simulink model "mcb_pmsm_foc_host_model_f28379d"  (R2023b)
settings: Solver=FixedStepDiscrete  StartTime=0.0  StopTime=inf  RelTol=1e-3  EnableMultiTasking=on
values from neighbouring files (symbols this model uses):
  dataType = 'single'    [mcb_pmsm_foc_sensorless_f28379d_datascript.m]    (also in mcb_pmsm_foc_test_f28379d_data.m)
  PU_System = mcb_SetPUSystem(pmsm,inverter)    [mcb_pmsm_foc_sensorless_f28379d_datascript.m]    (also in mcb_pmsm_foc_test_f28379d_data.m)
  Ts = T_pwm    [discrete_tansfer_fcn.m]    (also in mcb_pmsm_foc_sensorless_f28379d_datascript.m = 5e-05; mcb_pmsm_foc_test_f28379d_data.m = 5e-05)
libraries: instrumentseriallib x4, simulink x3
settings Model: Creator=The MathWorks, Inc.  LastModifiedBy=13571
settings SolverCC: AlgebraicLoopSolver=TrustRegion  MaxZcPerStep=1
settings DataIOCC: LimitDataPoints=on  SaveFormat=Array  ReturnWorkspaceOutputs=off
settings OptimizationCC: ReuseModelBlockBuffer=off  LifeSpan=1  EfficientTunableParamExpr=on
settings DebuggingCC: UnderspecifiedInitializationDetection=Classic  MergeDetectMultiDrivingBlocksExec=none  SolverPrmCheckMsg=warning  ParameterPrecisionLossMsg=none  UnconnectedInputMsg=warning  UnconnectedOutputMsg=warning  UnconnectedLineMsg=warning  AllowSymbolicDim=off  PregeneratedLibrarySubsystemCodeDiagnostic=none  SFUnexpectedBacktrackingDiag=warning  SFNoUnconditionalDefaultTransitionDiag=warning  SFExecutionAtInitializationDiag=none  ArithmeticOperatorsInVariantConditions=warning
settings HardwareCC: ProdBitPerPointer=32  ProdLargestAtomicFloat=None  ProdIntDivRoundTo=Undefined  ProdEndianess=Unspecified  ProdWordSize=32  ProdHWDeviceType=32-bit Generic
settings ModelReferenceCC: EnableRefExpFcnMdlSchedulingChecks=on  PropagateSignalLabelsOutOfModel=off
settings SFSimCC: SimUseLocalCustomCode=off  MATLABDynamicMemAlloc=off
settings RTWCC: Description=Real-Time Workshop Embedded Coder  SystemTargetFile=ert.tlc  TemplateMakefile=ert_default_tmf  GenerateReport=on  RTWUseLocalCustomCode=off  IncludeHyperlinkInReport=on  LaunchReport=on  GenerateTraceInfo=on  GenerateTraceReport=on  GenerateTraceReportSl=on  GenerateTraceReportSf=on  GenerateTraceReportEml=on  DLArmComputeVersion=19.05
settings CodeAppCC: IgnoreCustomStorageClasses=off  StateflowObjectComments=on  InternalIdentifier=Classic
settings ERTTargetCC: MultiwordLength=2048  GenerateSampleERTMain=on  ERTCustomFileTemplate=example_file_process.tlc  ConvertIfToSwitch=off  SuppressUnreachableDefaultCases=off
settings ConfigComp: CovMetricSettings=dw  CovSaveCumulativeToWorkspaceVar=on  CovSaveSingleToWorkspaceVar=on  CovExternalEMLEnable=off  CovSFcnEnable=off

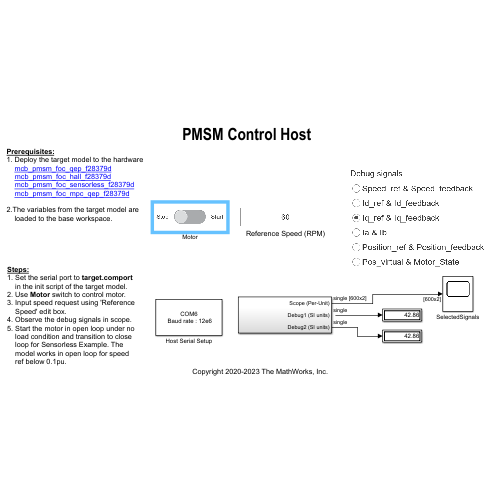
[thumbnail: Simulink's stored preview of the top-level diagram]
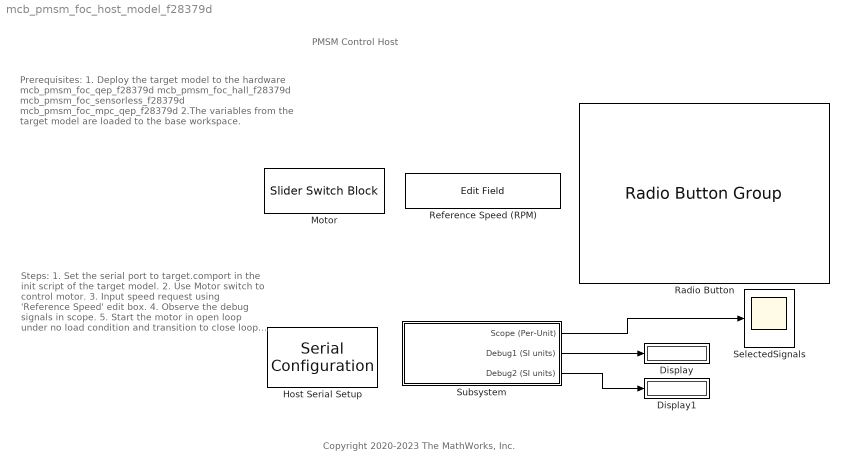
== system mcb_pmsm_foc_host_model_f28379d ==
  note: PMSM Control Host
  note: Copyright 2020-2023 The MathWorks, Inc.
  note: Steps:
      | 1. Set the serial port to target.comport
      | in the init script of the target model.
      | 2. Use Motor switch to control motor.
      | 3. Input speed request using 'Reference
      | Speed' edit box.
      | 4. Observe the debug signals in scope.
      | 5. Start the motor in open loop under no
      | load condition and transition to close
      | loop for Sensorless Example. The
      | model works in open loop for speed
      | ref below 0.1pu.
  note: Prerequisites:
      | 1. Deploy the target model to the hardware
      | mcb_pmsm_foc_qep_f28379d
      | mcb_pmsm_foc_hall_f28379d
      | mcb_pmsm_foc_sensorless_f28379d
      | mcb_pmsm_foc_mpc_qep_f28379d
      |
      | 2.The variables from the target model are
      | loaded to the base workspace.
  Display : Display
  Display1 : Display
  Host Serial Setup : instrumentseriallib/Serial Configuration  Priority=-99  PortSel=COM6  Port=COM6  ComPort=COM6  BaudRate=12e6  DataBits=8  Parity=none  StopBits=1  ByteOrder=little-endian  FlowControl=none  Timeout=2  SimulateUsing=Interpreted execution  BlockInModel=on  aMode=5
  Motor : SliderSwitchBlock  LabelPosition=Hide
      settings: Values={{'Stop', 'Start'}, [0 1]}
  Radio Button : RadioButtonGroup  LabelPosition=Hide  SelectedLabel=Iq_ref & Iq_feedback  ButtonGroupName=Debug signals
      settings: Values={{'Speed_ref & Speed_feedback', 'Id_ref & Id_feedback', 'Iq_ref & Iq_feedback', 'Ia & Ib', 'Position_ref & Position_feedback', 'Pos_virtual & Motor_State'}, [1 2 3 4 5 6]}
  Reference Speed (RPM) : EditField  LabelPosition=Hide  ShowInitialText=on  Alignment=Center
  SelectedSignals : Scope
  Subsystem : Subsystem
  wires:
  Subsystem/1(Scope (Per-Unit)) -> SelectedSignals/1
  Subsystem/2(Debug1 (SI units)) -> Display/1
  Subsystem/3(Debug2 (SI units)) -> Display1/1

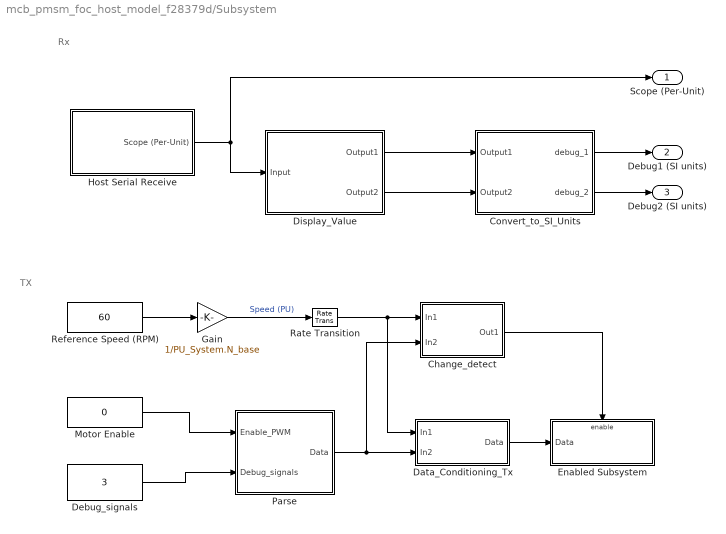
== system mcb_pmsm_foc_host_model_f28379d/Subsystem ==
  note: Rx
  note: TX
  Change_detect : Subsystem
  Convert_to_SI_Units : Subsystem
  Data_Conditioning_Tx : Subsystem  Variant=on
  Debug_signals : Constant  Value=3  OutDataTypeStr=uint16  SampleTime=0.03
  Display_Value : MATLAB Function  TreatAsAtomicUnit=on
  Enabled Subsystem : Subsystem  TreatAsAtomicUnit=on
  Gain : Gain  Gain=1/PU_System.N_base  RndMeth=Simplest  OutDataTypeStr=Inherit: Same as input
  Host Serial Receive : Subsystem  Variant=on
  Motor Enable : Constant  Value=0  VectorParams1D=off  OutDataTypeStr=uint16  SampleTime=0.03
  Parse : Subsystem
  Rate Transition : RateTransition  OutPortSampleTime=0.03
  Reference Speed (RPM) : Constant  Value=60  VectorParams1D=off  OutDataTypeStr=single  SampleTime=0.03
  Scope (Per-Unit) : Outport
  Debug1 (SI units) : Outport  Port=2
  Debug2 (SI units) : Outport  Port=3
  wires:
  Motor Enable/1 -> Parse/1(Enable_PWM)
  Change_detect/1(Out1) -> Enabled Subsystem/Enable
  Reference Speed (RPM)/1 -> Gain/1
  Rate Transition/1 -> Data_Conditioning_Tx/1(In1), Change_detect/1(In1)
  Parse/1(Data) -> Data_Conditioning_Tx/2(In2), Change_detect/2(In2)
  Data_Conditioning_Tx/1(Data) -> Enabled Subsystem/1(Data)
  Gain/1 -> Rate Transition/1  "Speed (PU)"
  Debug_signals/1 -> Parse/2(Debug_signals)
  Display_Value/2(Output2) -> Convert_to_SI_Units/2(Output2)
  Display_Value/1(Output1) -> Convert_to_SI_Units/1(Output1)
  Convert_to_SI_Units/2(debug_2) -> Debug2 (SI units)/1
  Convert_to_SI_Units/1(debug_1) -> Debug1 (SI units)/1
  Host Serial Receive/1(Scope (Per-Unit)) -> Scope (Per-Unit)/1, Display_Value/1(Input)

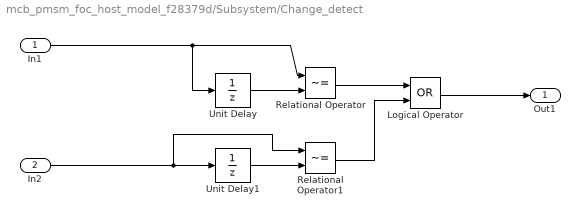
== system mcb_pmsm_foc_host_model_f28379d/Subsystem/Change_detect ==
  In1 : Inport
  In2 : Inport  Port=2
  Logical Operator : Logic  Operator=OR  AllPortsSameDT=off  OutDataTypeStr=boolean
  Relational Operator : RelationalOperator  Operator=~=  OutDataTypeStr=boolean  InputSameDT=off
  Relational Operator1 : RelationalOperator  Operator=~=  OutDataTypeStr=boolean  InputSameDT=off
  Unit Delay : UnitDelay  InitialCondition=0.5  SampleTime=-1  HasFrameUpgradeWarning=on
  Unit Delay1 : UnitDelay  SampleTime=-1  HasFrameUpgradeWarning=on
  Out1 : Outport  VectorParamsAs1DForOutWhenUnconnected=off
  wires:
  In2/1 -> Relational Operator1/1, Unit Delay1/1
  Relational Operator1/1 -> Logical Operator/2
  Unit Delay1/1 -> Relational Operator1/2
  Unit Delay/1 -> Relational Operator/2
  In1/1 -> Unit Delay/1, Relational Operator/1
  Relational Operator/1 -> Logical Operator/1
  Logical Operator/1 -> Out1/1

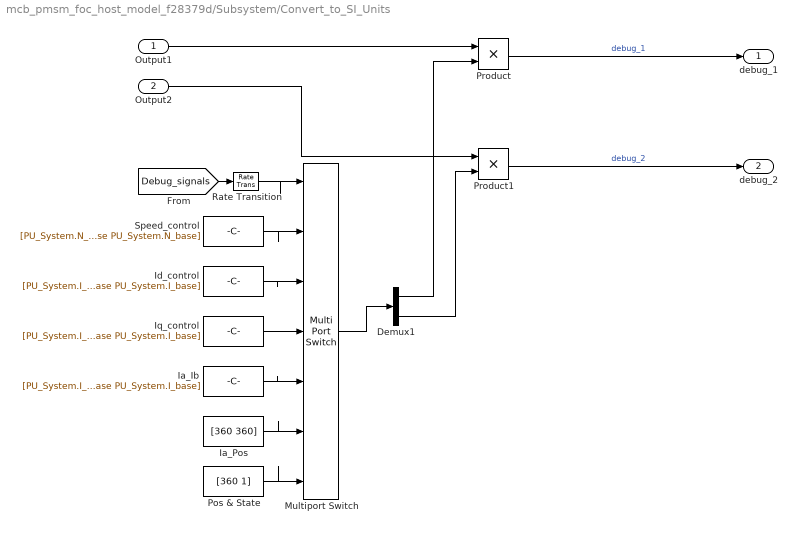
== system mcb_pmsm_foc_host_model_f28379d/Subsystem/Convert_to_SI_Units ==
  Output1 : Inport
  Output2 : Inport  Port=2
  Demux1 : Demux  Outputs=2
  Ia_Ib : Constant  Value=[PU_System.I_base PU_System.I_base]  OutDataTypeStr=single  SampleTime=-1
  Ia_Pos : Constant  Value=[360 360]  OutDataTypeStr=single  SampleTime=-1
  Id_control : Constant  Value=[PU_System.I_base PU_System.I_base]  OutDataTypeStr=single  SampleTime=-1
  Iq_control : Constant  Value=[PU_System.I_base PU_System.I_base]  OutDataTypeStr=single  SampleTime=-1
  Multiport Switch : MultiPortSwitch  Inputs=6  DiagnosticForDefault=Warning  OutDataTypeStr=single  RndMeth=Simplest  SaturateOnIntegerOverflow=off  InputSameDT=off
  Pos & State : Constant  Value=[360 1]  OutDataTypeStr=single  SampleTime=-1
  Product : Product
  Product1 : Product
  Rate Transition : RateTransition  Deterministic=off
  Speed_control : Constant  Value=[PU_System.N_base PU_System.N_base]  OutDataTypeStr=single  SampleTime=-1
  debug_1 : Outport
  debug_2 : Outport  Port=2
  wires:
  Product/1 -> debug_1/1  "debug_1"
  Product1/1 -> debug_2/1  "debug_2"
  [Debug_signals] -> Rate Transition/1
  Id_control/1 -> Multiport Switch/3
  Speed_control/1 -> Multiport Switch/2
  Multiport Switch/1 -> Demux1/1
  Ia_Ib/1 -> Multiport Switch/5
  Iq_control/1 -> Multiport Switch/4
  Demux1/2 -> Product1/2
  Demux1/1 -> Product/2
  Ia_Pos/1 -> Multiport Switch/6
  Output1/1 -> Product/1
  Output2/1 -> Product1/1
  Rate Transition/1 -> Multiport Switch/1
  Pos & State/1 -> Multiport Switch/7

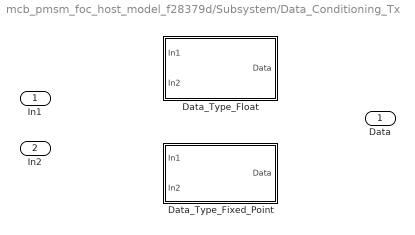
== system mcb_pmsm_foc_host_model_f28379d/Subsystem/Data_Conditioning_Tx ==
  In1 : Inport
  In2 : Inport  Port=2
  Data_Type_Fixed_Point : Subsystem  VariantControl=~isequal(dataType, 'single')
  Data_Type_Float : Subsystem  VariantControl=isequal(dataType, 'single')
  Data : Outport

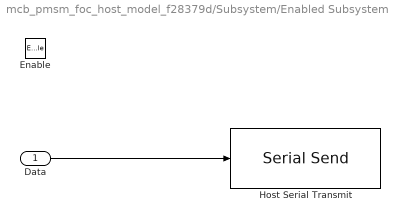
== system mcb_pmsm_foc_host_model_f28379d/Subsystem/Enabled Subsystem ==
  Data : Inport
  Enable : EnablePort
  Host Serial Transmit : instrumentseriallib/Serial Send  PortSel=COM6  Port=COM6  ComPort=COM6  Header=[]  Terminator=<none>  CustomTerminator=[]  EnableBlockingMode=off  SimulateUsing=Interpreted execution  BlockInModel=on  aMode=5
  wires:
  Data/1 -> Host Serial Transmit/1

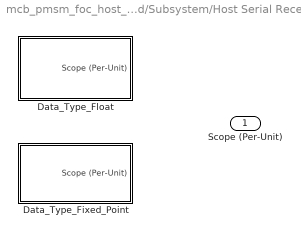
== system mcb_pmsm_foc_host_model_f28379d/Subsystem/Host Serial Receive ==
  Data_Type_Fixed_Point : Subsystem  VariantControl=~isequal(dataType, 'single')
  Data_Type_Float : Subsystem  VariantControl=isequal(dataType, 'single')
  Scope (Per-Unit) : Outport

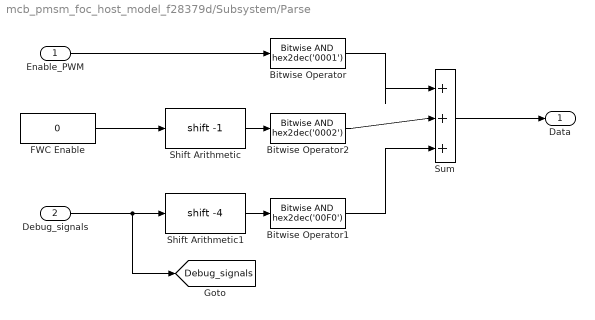
== system mcb_pmsm_foc_host_model_f28379d/Subsystem/Parse ==
  Enable_PWM : Inport
  Debug_signals : Inport  Port=2
  Bitwise Operator : simulink/Logic and Bit Operations/Bitwise Operator  logicop=AND  UseBitMask=on  BitMask=hex2dec('0001')  BitMaskRealWorld=Stored Integer
  Bitwise Operator1 : simulink/Logic and Bit Operations/Bitwise Operator  logicop=AND  UseBitMask=on  BitMask=hex2dec('00F0')  BitMaskRealWorld=Stored Integer
  Bitwise Operator2 : simulink/Logic and Bit Operations/Bitwise Operator  logicop=AND  UseBitMask=on  BitMask=hex2dec('0002')  BitMaskRealWorld=Stored Integer
  FWC Enable : Constant  Value=0  VectorParams1D=off  OutDataTypeStr=uint16  SampleTime=0.03
  Shift Arithmetic : ArithShift  BitShiftNumber=-1
  Shift Arithmetic1 : ArithShift  BitShiftNumber=-4
  Sum : Sum  Inputs=|+++
  Data : Outport
  tag scope: Debug_signals=global
  wires:
  Bitwise Operator/1 -> Sum/1
  Debug_signals/1 -> [Debug_signals], Shift Arithmetic1/1
  Sum/1 -> Data/1
  Shift Arithmetic1/1 -> Bitwise Operator1/1
  Shift Arithmetic/1 -> Bitwise Operator2/1
  Bitwise Operator1/1 -> Sum/3
  FWC Enable/1 -> Shift Arithmetic/1
  Bitwise Operator2/1 -> Sum/2
  Enable_PWM/1 -> Bitwise Operator/1

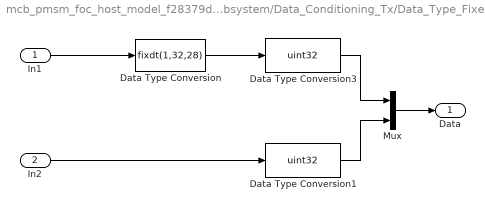
== system mcb_pmsm_foc_host_model_f28379d/Subsystem/Data_Conditioning_Tx/Data_Type_Fixed_Point ==
  In1 : Inport
  In2 : Inport  Port=2
  Data Type Conversion : DataTypeConversion  OutDataTypeStr=fixdt(1,32,28)  RndMeth=Simplest  SaturateOnIntegerOverflow=off
  Data Type Conversion1 : DataTypeConversion  OutDataTypeStr=uint32  RndMeth=Simplest  SaturateOnIntegerOverflow=off
  Data Type Conversion3 : DataTypeConversion  OutDataTypeStr=uint32  ConvertRealWorld=Stored Integer (SI)  RndMeth=Simplest  SaturateOnIntegerOverflow=off
  Mux : Mux  Inputs=2
  Data : Outport
  wires:
  In1/1 -> Data Type Conversion/1
  Data Type Conversion3/1 -> Mux/1
  Data Type Conversion/1 -> Data Type Conversion3/1
  In2/1 -> Data Type Conversion1/1
  Data Type Conversion1/1 -> Mux/2
  Mux/1 -> Data/1

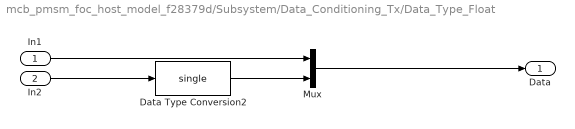
== system mcb_pmsm_foc_host_model_f28379d/Subsystem/Data_Conditioning_Tx/Data_Type_Float ==
  In1 : Inport
  In2 : Inport  Port=2
  Data Type Conversion2 : DataTypeConversion  OutDataTypeStr=single  RndMeth=Simplest  SaturateOnIntegerOverflow=off
  Mux : Mux  Inputs=2
  Data : Outport
  wires:
  In1/1 -> Mux/1
  Mux/1 -> Data/1
  In2/1 -> Data Type Conversion2/1
  Data Type Conversion2/1 -> Mux/2

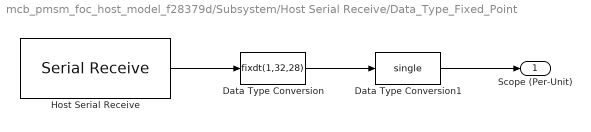
== system mcb_pmsm_foc_host_model_f28379d/Subsystem/Host Serial Receive/Data_Type_Fixed_Point ==
  Data Type Conversion : DataTypeConversion  OutDataTypeStr=fixdt(1,32,28)  ConvertRealWorld=Stored Integer (SI)  RndMeth=Simplest  SaturateOnIntegerOverflow=off
  Data Type Conversion1 : DataTypeConversion  OutDataTypeStr=single  RndMeth=Simplest  SaturateOnIntegerOverflow=off
  Host Serial Receive : instrumentseriallib/Serial Receive  PortSel=target.comport  Port=target.comport  ComPort=target.comport  DataType=uint32  SaveDataType=uint8  ToggleHeader=on  Header='SSSS'  ToggleTerminator=on  Terminator=Custom terminator  CustomTerminator='EEEE'  InputFormat=Row major  ToggleDataSize=on  DataSize=[600 2]  EnableBlockingMode=on  ActionDataUnavailable=Output custom value  ActionWhenDataUnavailable=Output custom value  CustomValue=4  SampleTime=600*Ts  SimulateUsing=Interpreted execution  BlockInModel=on  aMode=5
  Scope (Per-Unit) : Outport
  wires:
  Data Type Conversion/1 -> Data Type Conversion1/1
  Host Serial Receive/1 -> Data Type Conversion/1
  Data Type Conversion1/1 -> Scope (Per-Unit)/1

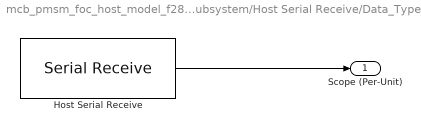
== system mcb_pmsm_foc_host_model_f28379d/Subsystem/Host Serial Receive/Data_Type_Float ==
  Host Serial Receive : instrumentseriallib/Serial Receive  PortSel=COM6  Port=COM6  ComPort=COM6  DataType=single  SaveDataType=uint8  ToggleHeader=on  Header='SSSS'  DataSize=[600 2]  ToggleTerminator=on  Terminator=Custom terminator  CustomTerminator='EEEE'  InputFormat=Row major  ToggleDataSize=on  EnableBlockingMode=on  ActionDataUnavailable=Output custom value  ActionWhenDataUnavailable=Output custom value  CustomValue=4  SampleTime=600*Ts  SimulateUsing=Interpreted execution  BlockInModel=on  aMode=5
  Scope (Per-Unit) : Outport
  wires:
  Host Serial Receive/1 -> Scope (Per-Unit)/1

== matlab function mcb_pmsm_foc_host_model_f28379d/Subsystem/Display_Value ==
  data: Output1 output; Output2 output; Input input
function [ Output1, Output2] = unBuf(Input)
% Unbuffer function
% Outputs first received serial data from buffer for both signals

% Copyright 2020 The MathWorks, Inc.

selSignal= Input(:, 1);
Output1 = selSignal(1,1);
selSignal = Input(:, 2);
Output2 = selSignal(1,1);
end
